simulink model "InverseKinematics"  (R2021a)
settings: Solver=VariableStepAuto  StartTime=0.0  StopTime=inf  RelTol=1e-3
settings Model: Creator=Al ien  LastModifiedBy=Al ien

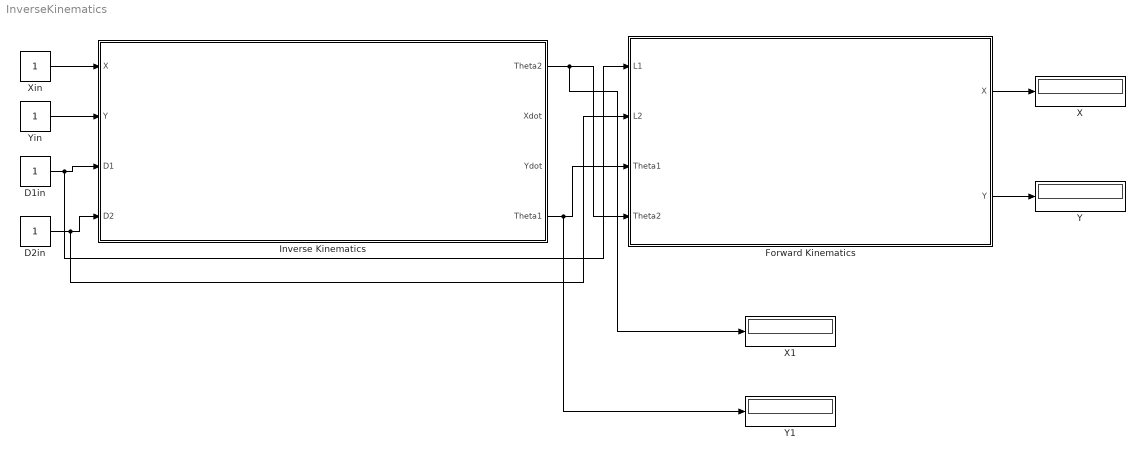
== system InverseKinematics ==
  D1in : Constant
  D2in : Constant
  Forward Kinematics : Subsystem
  Inverse Kinematics : Subsystem
  X : Display
  X1 : Display
  Xin : Constant
  Y : Display
  Y1 : Display
  Yin : Constant
  wires:
  Inverse Kinematics/1(Theta2) -> X1/1, Forward Kinematics/4(Theta2)
  Inverse Kinematics/4(Theta1) -> Y1/1, Forward Kinematics/3(Theta1)
  Forward Kinematics/1(X) -> X/1
  Forward Kinematics/2(Y) -> Y/1
  Yin/1 -> Inverse Kinematics/2(Y)
  Xin/1 -> Inverse Kinematics/1(X)
  D1in/1 -> Forward Kinematics/1(L1), Inverse Kinematics/3(D1)
  D2in/1 -> Forward Kinematics/2(L2), Inverse Kinematics/4(D2)

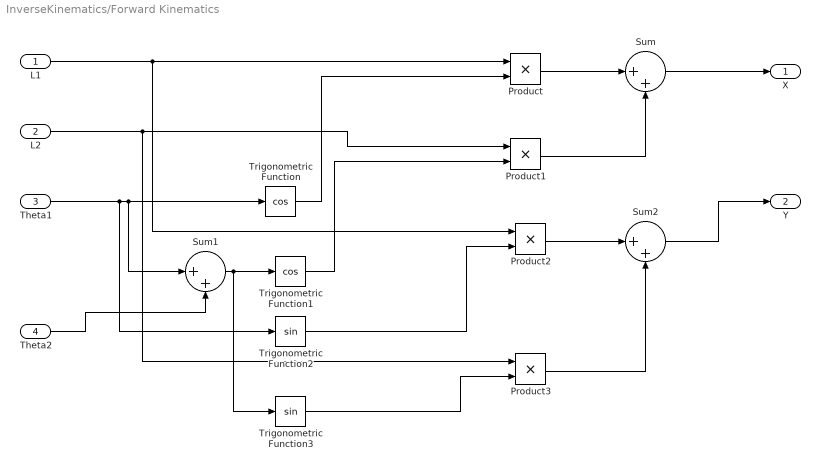
== system InverseKinematics/Forward Kinematics ==
  L1 : Inport
  L2 : Inport  Port=2
  Theta1 : Inport  Port=3
  Theta2 : Inport  Port=4
  Product{,1..3} (4 alike) : Product
  Sum : Sum  Inputs=|++
  Sum1 : Sum  Inputs=|++
  Sum2 : Sum  Inputs=|++
  Trigonometric Function : Trigonometry  Operator=cos
  Trigonometric Function1 : Trigonometry  Operator=cos
  Trigonometric Function2 : Trigonometry
  Trigonometric Function3 : Trigonometry
  X : Outport
  Y : Outport  Port=2
  wires:
  L1/1 -> Product2/1, Product/1
  Theta1/1 -> Trigonometric Function2/1, Sum1/1, Trigonometric Function/1
  Product2/1 -> Sum2/1
  Trigonometric Function1/1 -> Product1/2
  L2/1 -> Product3/1, Product1/1
  Sum2/1 -> Y/1
  Product/1 -> Sum/1
  Sum1/1 -> Trigonometric Function3/1, Trigonometric Function1/1
  Theta2/1 -> Sum1/2
  Trigonometric Function3/1 -> Product3/2
  Product1/1 -> Sum/2
  Trigonometric Function2/1 -> Product2/2
  Sum/1 -> X/1
  Trigonometric Function/1 -> Product/2
  Product3/1 -> Sum2/2

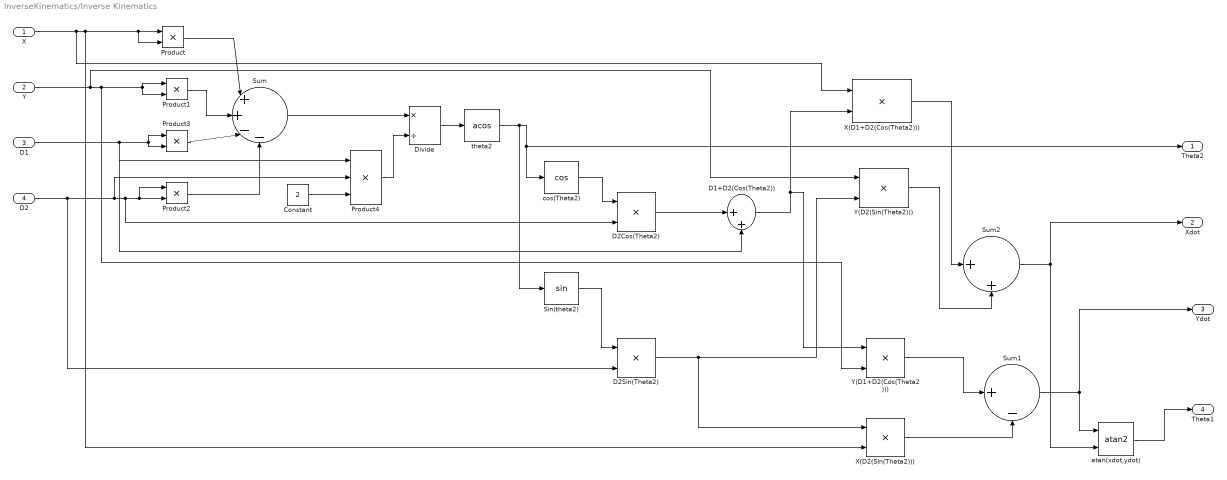
== system InverseKinematics/Inverse Kinematics ==
  X : Inport
  Y : Inport  Port=2
  D1 : Inport  Port=3
  D2 : Inport  Port=4
  Constant : Constant  Value=2
  D1+D2(Cos(Theta2)) : Sum  Inputs=|++
  D2Cos(Theta2) : Product
  D2Sin(Theta2) : Product
  Divide : Product  Inputs=*/
  Product{,1..3} (4 alike) : Product
  Product4 : Product  Inputs=3
  Sin(theta2) : Trigonometry
  Sum : Sum  Inputs=|++--
  Sum1 : Sum  Inputs=|+-
  Sum2 : Sum  Inputs=|++
  X(D1+D2(Cos(Theta2))) : Product
  X(D2(Sin(Theta2))) : Product
  Y(D1+D2(Cos(Theta2))) : Product
  Y(D2(Sin(Theta2))) : Product
  atan(xdot,ydot) : Trigonometry  Operator=atan2
  cos(Theta2) : Trigonometry  Operator=cos
  theta2 : Trigonometry  Operator=acos
  Theta2 : Outport
  Xdot : Outport  Port=2
  Ydot : Outport  Port=3
  Theta1 : Outport  Port=4
  wires:
  D2Sin(Theta2)/1 -> X(D2(Sin(Theta2)))/1, Y(D2(Sin(Theta2)))/2
  Product1/1 -> Sum/2
  Sum/1 -> Divide/1
  Divide/1 -> theta2/1
  Product/1 -> Sum/1
  Sin(theta2)/1 -> D2Sin(Theta2)/1
  D1+D2(Cos(Theta2))/1 -> Y(D1+D2(Cos(Theta2)))/1, X(D1+D2(Cos(Theta2)))/2
  Product4/1 -> Divide/2
  Product3/1 -> Sum/3
  Y(D2(Sin(Theta2)))/1 -> Sum2/2
  Y(D1+D2(Cos(Theta2)))/1 -> Sum1/1
  D1/1 -> D1+D2(Cos(Theta2))/2, Product3/2, Product3/1, Product4/1
  D2/1 -> D2Sin(Theta2)/2, Product4/2, D2Cos(Theta2)/2, Product2/1, Product2/2
  X/1 -> X(D1+D2(Cos(Theta2)))/1, X(D2(Sin(Theta2)))/2, Product/2, Product/1
  Sum1/1 -> Ydot/1, atan(xdot,ydot)/1
  cos(Theta2)/1 -> D2Cos(Theta2)/1
  Sum2/1 -> Xdot/1, atan(xdot,ydot)/2
  X(D2(Sin(Theta2)))/1 -> Sum1/2
  theta2/1 -> Sin(theta2)/1, Theta2/1, cos(Theta2)/1
  Y/1 -> Y(D2(Sin(Theta2)))/1, Y(D1+D2(Cos(Theta2)))/2, Product1/1, Product1/2
  X(D1+D2(Cos(Theta2)))/1 -> Sum2/1
  D2Cos(Theta2)/1 -> D1+D2(Cos(Theta2))/1
  Product2/1 -> Sum/4
  Constant/1 -> Product4/3
  atan(xdot,ydot)/1 -> Theta1/1
